simulink library "coeff_gen_lib"  (Simulink 6.2)
libraries: xbsIndex_r3 x12, coeff_gen_lib x1
settings Model: LastModifiedBy=aparsons

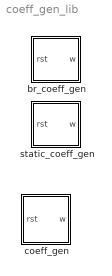
== system coeff_gen_lib ==
  br_coeff_gen : Subsystem  mask{Coeffs=[0 1 2 3], StepPeriod=0, n_bits=18, latency=4}
      mask prompts: Coeffs "Coefficients: (0 to 2^(FFTSize-1)-1)"; StepPeriod "Step Period: (2^?)"; n_bits "Bit Width:"
      mask init:
      | cursys = gcb;
      | disp(cursys);
      | vlen = length(Coeffs);
  coeff_gen : Subsystem  BlockChoice=br_coeff_gen
      settings: TemplateBlock=self  MemberBlocks=br_coeff_gen,static_coeff_gen
  static_coeff_gen : Subsystem  mask{Coeffs=0, n_bits=18, latency=4}
      mask prompts: Coeffs "Coefficients: (0 to 2^(FFTSize-1)-1)"; n_bits "Bit Width:"
      mask init:
      | cursys = gcb;
      | disp(cursys);

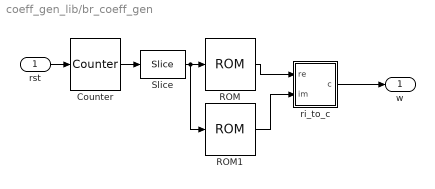
== system coeff_gen_lib/br_coeff_gen ==
  rst : Inport  Port=1  LatchInput=off
  Counter : xbsIndex_r3/Counter  cnt_type=Free Running  n_bits=log2(vlen) + StepPeriod  bin_pt=0  arith_type=Unsigned  start_count=0  cnt_to=Inf  cnt_by_val=1  operation=Up  explicit_period=off  period=1  load_pin=off  rst=on  en=off  dbl_ovrd=off  show_param=off  use_rpm=on  gen_core=off
      settings: xl_area=[0, 0, 0, 0, 0, 0, 0]
  ROM : xbsIndex_r3/ROM  depth=vlen  initVector=round( real(Coeffs) * 2^(n_bits-1) ) / 2^(n_bits-1)  arith_type="Signed  (2's comp)"  n_bits=n_bits  bin_pt=n_bits-1  latency=latency  init_zero=on  explicit_period=off  period=1  rst=off  init_reg=0  en=off  dbl_ovrd=off  show_param=on  distributed_mem=on  use_rpm=off  gen_core=off
      settings: xl_area=[0, 0, 0, 0, 0, 0, 0]
  ROM1 : xbsIndex_r3/ROM  depth=vlen  initVector="round( imag(Coeffs) * 2^(n_bits-1)  ) / 2^(n_bits-1)"  arith_type="Signed  (2's comp)"  n_bits=n_bits  bin_pt=n_bits-1  latency=latency  init_zero=on  explicit_period=off  period=1  rst=off  init_reg=0  en=off  dbl_ovrd=off  show_param=on  distributed_mem=on  use_rpm=off  gen_core=off
      settings: xl_area=[0, 0, 0, 0, 0, 0, 0]
  Slice : xbsIndex_r3/Slice  mode=Upper Bit Location + Width  nbits=log2(vlen)  bit1=0  base1=MSB of Input  bit0=0  base0=LSB of Input  boolean_output=off  explicit_period=off  period=1  dbl_ovrd=off
  ri_to_c : Subsystem
  w : Outport
  wires:
  ri_to_c/1(c) -> w/1
  ROM1/1 -> ri_to_c/2(im)
  ROM/1 -> ri_to_c/1(re)
  Slice/1 -> ROM1/1, ROM/1
  rst/1 -> Counter/1
  Counter/1 -> Slice/1

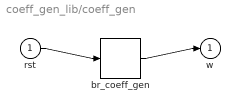
== system coeff_gen_lib/coeff_gen ==
  rst : Inport  Port=1  LatchInput=off
  br_coeff_gen : coeff_gen_lib/br_coeff_gen  Coeffs=[0 1 2 3]  StepPeriod=0  n_bits=18  latency=4
  w : Outport
  wires:
  rst/1 -> br_coeff_gen/1
  br_coeff_gen/1 -> w/1

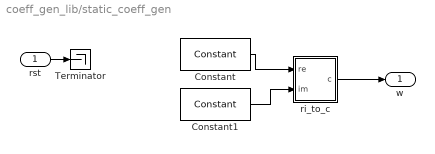
== system coeff_gen_lib/static_coeff_gen ==
  rst : Inport  Port=1  LatchInput=off
  Constant : xbsIndex_r3/Constant  const=round(real(Coeffs(1)) * 2^(n_bits-1)) / 2^(n_bits-1)  equ=P=C  arith_type="Signed  (2's comp)"  n_bits=n_bits  bin_pt=n_bits - 1  opselect=C  inp2=PCIN>>17  opr=+  inp1=P  carry=CIN  iostate=0  explicit_period=on  period=1  dbl_ovrd=off
  Constant1 : xbsIndex_r3/Constant  const=round(imag(Coeffs(1)) * 2^(n_bits-1)) / 2^(n_bits-1)  equ=P=C  arith_type="Signed  (2's comp)"  n_bits=n_bits  bin_pt=n_bits - 1  opselect=C  inp2=PCIN>>17  opr=+  inp1=P  carry=CIN  iostate=0  explicit_period=on  period=1  dbl_ovrd=off
  Terminator : Terminator
  ri_to_c : Subsystem
  w : Outport
  wires:
  rst/1 -> Terminator/1
  Constant/1 -> ri_to_c/1(re)
  Constant1/1 -> ri_to_c/2(im)
  ri_to_c/1(c) -> w/1

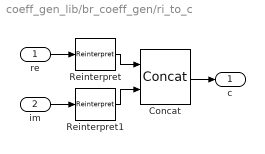
== system coeff_gen_lib/br_coeff_gen/ri_to_c ==
  re : Inport  Port=1  LatchInput=off
  im : Inport  Port=2  LatchInput=off
  Concat : xbsIndex_r3/Concat  num_inputs=2  explicit_period=off  period=1  dbl_ovrd=off
  Reinterpret : xbsIndex_r3/Reinterpret  force_arith_type=on  arith_type=Unsigned  force_bin_pt=on  bin_pt=0  force_valid=on
  Reinterpret1 : xbsIndex_r3/Reinterpret  force_arith_type=on  arith_type=Unsigned  force_bin_pt=on  bin_pt=0  force_valid=on
  c : Outport
  wires:
  im/1 -> Reinterpret1/1
  Concat/1 -> c/1
  re/1 -> Reinterpret/1
  Reinterpret1/1 -> Concat/2
  Reinterpret/1 -> Concat/1

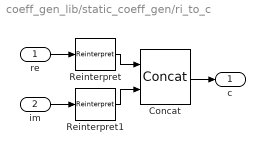
== system coeff_gen_lib/static_coeff_gen/ri_to_c ==
  re : Inport  Port=1  LatchInput=off
  im : Inport  Port=2  LatchInput=off
  Concat : xbsIndex_r3/Concat  num_inputs=2  explicit_period=off  period=1  dbl_ovrd=off
  Reinterpret : xbsIndex_r3/Reinterpret  force_arith_type=on  arith_type=Unsigned  force_bin_pt=on  bin_pt=0  force_valid=on
  Reinterpret1 : xbsIndex_r3/Reinterpret  force_arith_type=on  arith_type=Unsigned  force_bin_pt=on  bin_pt=0  force_valid=on
  c : Outport
  wires:
  im/1 -> Reinterpret1/1
  Concat/1 -> c/1
  re/1 -> Reinterpret/1
  Reinterpret1/1 -> Concat/2
  Reinterpret/1 -> Concat/1
